simulink model "sl_interactions"  (R2017b)
settings: Solver=FixedStepAuto  StartTime=0.0  StopTime=10.0  RelTol=1e-3  EnableMultiTasking=on
undefined symbols (not defined in the file or in its folder): params
libraries: simulink x1
settings Model: Creator=na364  LastModifiedBy=na364
settings DataIOCC: LimitDataPoints=on
settings OptimizationCC: LifeSpan=inf
settings DebuggingCC: AllowSymbolicDim=off  SFUnexpectedBacktrackingDiag=warning  SFNoUnconditionalDefaultTransitionDiag=warning  SFExecutionAtInitializationDiag=none
settings ModelReferenceCC: PropagateSignalLabelsOutOfModel=off
settings CodeAppCC: StateflowObjectComments=on
settings GRTTargetCC: TargetLangStandard=C89/C90 (ANSI)
settings ConfigComp: CovMetricSettings=dw  CovHtmlReporting=on  CovSaveCumulativeToWorkspaceVar=on  CovSaveSingleToWorkspaceVar=on  CovExternalEMLEnable=off

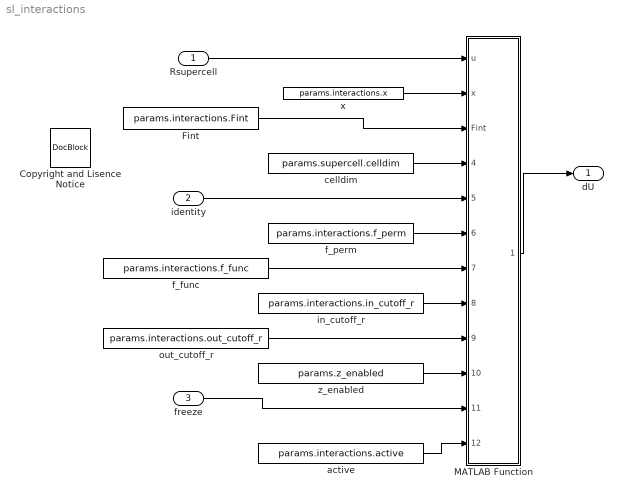
== system sl_interactions ==
  Rsupercell : Inport  PortDimensions=[params.model_dim,params.Nprtcl]
  identity : Inport  Port=2  PortDimensions=[1,params.Nprtcl]
  freeze : Inport  Port=3  PortDimensions=[1,params.Nprtcl]
  Copyright and Lisence Notice : simulink/Model-Wide Utilities/DocBlock  DocumentType=Text
      content=|
      | % Copyright (c) 2018, Nadav Avidor.
      | % All rights reserved.
      | % This file is part of the PIGLE - Particles Interacting in Generalized Langevin Equation simulator, subject to the
      | % GNU/GPL-3.0-or-later.
  Fint : Constant  Value=params.interactions.Fint
  MATLAB Function : MATLAB Function  TreatAsAtomicUnit=on
  active : Constant  Value=params.interactions.active
  celldim : Constant  Value=params.supercell.celldim
  f_func : Constant  Value=params.interactions.f_func
  f_perm : Constant  Value=params.interactions.f_perm
  in_cutoff_r : Constant  Value=params.interactions.in_cutoff_r
  out_cutoff_r : Constant  Value=params.interactions.out_cutoff_r
  x : Constant  Value=params.interactions.x
  z_enabled : Constant  Value=params.z_enabled
  dU : Outport  PortDimensions=[params.model_dim,params.Nprtcl]
  wires:
  Rsupercell/1 -> MATLAB Function/1(u)
  celldim/1 -> MATLAB Function/4(celldim)
  Fint/1 -> MATLAB Function/3(Fint)
  x/1 -> MATLAB Function/2(x)
  identity/1 -> MATLAB Function/5(identity)
  f_perm/1 -> MATLAB Function/6(f_perm)
  f_func/1 -> MATLAB Function/7(f_func)
  in_cutoff_r/1 -> MATLAB Function/8(in_cutoff_r)
  out_cutoff_r/1 -> MATLAB Function/9(out_cutoff_r)
  z_enabled/1 -> MATLAB Function/10(z_enabled)
  MATLAB Function/1(Force_int) -> dU/1
  freeze/1 -> MATLAB Function/11(freeze)
  active/1 -> MATLAB Function/12(active)

== matlab function sl_interactions/MATLAB Function ==
  data: u input; Force_int output; x input; Fint input; celldim input; identity input; f_perm input; f_func input; in_cutoff_r input; out_cutoff_r input; z_enabled input; freeze input; active input
function Force_int   = Fij(u,x,Fint,celldim,identity,f_perm, f_func,in_cutoff_r,out_cutoff_r,z_enabled,freeze,active)

      Force_int = zeros(size(u));
      a = celldim(1)/2;
      b = celldim(2)/2;
      
      if size(x,1) < size(x,2)
          x=x';
      end
      if size(Fint,1) < size(Fint,2)
          Fint1 = Fint';
      else
          Fint1 = Fint;
      end
      
      nop = size(u,2);
      
      
      if ( nop > 1 && active )
          
          r =zeros(nop); R = zeros(nop); sin_phi = zeros(nop); cos_phi = zeros(nop);
          sine = zeros(nop); cosine = zeros(nop); f_indx = zeros(nop);
                
        for i = 1:1:nop
            if freeze(i) == 1, continue; end
              for j = i+1:1:nop
                  
                  if freeze(j) == 1, continue; end

                  % Interaction out of the various permutations
                  % TODO: The 9 following lines could be replaced probably with:
                  % perm = sum(bsxfun(@eq,sort([identity(i) identity(j)]),f_perm),2)==2;
                  perm1 = sum(bsxfun(@eq,[identity(i) identity(j)],f_perm),2)==2;
                  perm2 = sum(bsxfun(@eq,[identity(j) identity(i)],f_perm),2)==2;
                  if any(perm1)
                      perm = perm1;
                  elseif any(perm2)
                      perm = perm2;
                  else
                      error('Fij function: No such perm')
                  end                                       
                  
                  % For the j,i pair, which force function is to be used?
                  f_indx(j,i) = 0;
                  for permInd=1:length(perm)
                      if perm(permInd) > 0, f_indx(j,i) = permInd; end
                  end
                  %if f_indx(j,i) == 0, error(['permutation in (j,i)=' num2str([j i]) ' not assigned']); end
                  
                  %% Work out the distance between the pair of particles
                  
                  % Cartezian components of the distance (x,y,z)
                  if(abs(u(1,i)-u(1,j))>(a))
                      xeff = u(1,i)- u(1,j) - 2*a *  (u(1,i)- u(1,j))/abs(u(1,i)- u(1,j));
                  else
                      xeff = u(1,i) - u(1,j);
                  end
                  if(abs(u(2,i)-u(2,j))>(b))
                      yeff = u(2,i)- u(2,j) - 2*b *  (u(2,i)- u(2,j))/abs(u(2,i)- u(2,j));
                  else
                      yeff = u(2,i) - u(2,j);
                  end
                  
                  if z_enabled > 0 && size(u,1) > 2
                      zeff = u(3,i) - u(3,j);
                  else
                      zeff = 0;
                  end
                  
                  % Projection on the surface
                  R(j,i) = sqrt(xeff.^2 + yeff.^2);
                  sine(j,i) = yeff/R(j,i);
                  cosine(j,i) = xeff/R(j,i);
                  
                  % Total distance, and projection prependicular to the surface
                  r(j,i) = sqrt(R(j,i).^2 + zeff.^2);
                  cos_phi(j,i) = zeff/r(j,i);
                  sin_phi(j,i) = R(j,i)/r(j,i);
                  
                  % Do not allow particles to be too close (mainly can
                  % happen during init stage)
                  if r(j,i) < in_cutoff_r
                      r(j,i) = in_cutoff_r;
                  end
                      
              end
        end
        
        % Here the force for each pair of particle is calculated.
        % A long explanation with an example:
        % Assuming we have two populations P1 and P2 of particles,
        % different forces will (potentialy) act. f_perm holds all
        % the posible permutations, and for two populations it needs
        % to be defined as f_perm=[1 1; 1 2; 2 2]. We then need to
        % define force function for each permutation, and we do that
        % with f_func. f_func will then hold the function number
        % (case in the file  f_interactions.m) for each permutation, lets say f_func=[1,2,1],
        % which says that there is a power series like function between
        % 1-1 and 2-2, but zero force between particles from different
        % populations (1-2). so f_func(3) defines the force function to be
        % used for pairs of particles corresponding to f_perm(3) which [2
        % 2], ie cases were both particles are from population 2.
        % Fint1 is a matrix of the decimated forces, where Fint1(x,k) is
        % the decimated force for the permutation k (calculated with the function defined in f_func).
        
        % f_indx is a 2D matrix for the pair of particles (i,j), which
        % defines the permutation of each pair. So f_indx(i,j) holds the
        % row number in Fint1, which holds the decimated force to be used
        % for (i,j).
        
        Fs = zeros(nop);
        % For the number of permutations defined
        % [ size(f_perm,1) could be used insteed  ]
        for i=1:length(f_func)
            % Interpulate the force for all pairs of atoms assuming they belong to the
            % i'th permitatuon, but multiply with zero all the results
            % for pairs belonging to different permutation. [Sum on all
            % permutations]
            Fs= Fs + (f_indx==i) .* interp1(x,Fint1(:,i),r,'linear',0);
        end
        
        F_parall = Fs.*sin_phi;
        Fz = Fs.*cos_phi; Fz = Fz - Fz';
        
        % The forces acts on both particles in each pair of atoms, and we
        % have only worked out by now one triange in each force matrix.
        Fx = F_parall.*cosine; Fx = Fx - Fx';
        Fy = F_parall.*sine; Fy = Fy - Fy';
        
        for i = 1:1:nop
            Force_int(1,i) = sum(Fx(i,:));
            Force_int(2,i) = sum(Fy(i,:));
            if size(Force_int,1) > 2
                Force_int(3,i) = sum(Fz(i,:));
            end
        end
      end
      
end
